simulink subsystem "Bat_lookup_2024a"  (R2024a)
settings: Solver=VariableStepAuto  StartTime=0.0  StopTime=10.0  RelTol=1e-3
settings Model: Creator=User  LastModifiedBy=User

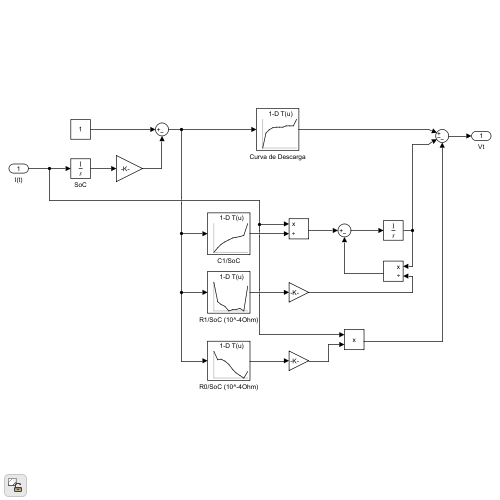
[thumbnail: Simulink's stored preview of the top-level diagram]
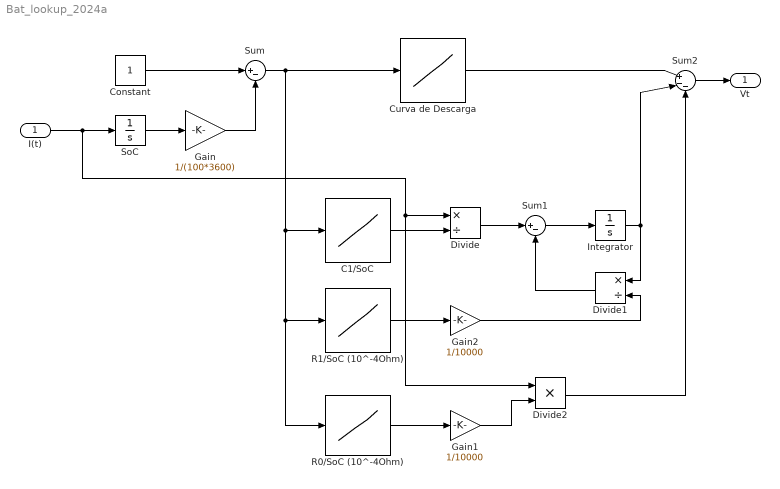
== system Bat_lookup_2024a ==
  I(t) : Inport
  C1/SoC : Lookup_n-D  NumberOfTableDimensions=1  BreakpointsForDimension1=[0.1;0.2;0.3;0.4;0.5;0.6;0.7;0.8;0.9;1]  Table=[14627;21365;25642;29230;32161;34533;36341;37291;38369;55644]  InternalRulePriority=Speed  RndMeth=Simplest
  Constant : Constant
  Curva de Descarga : Lookup_n-D  NumberOfTableDimensions=1  BreakpointsForDimension1=[0 0.10000000000000001 0.20000000000000001 0.29999999999999999 0.40000000000000002 0.5 0.59999999999999998 0.69999999999999996 0.80000000000000004 0.90000000000000002 1]  Table=[2.734 3.127 3.213 3.256 3.278 3.28 3.285 3.308 3.319 3.32 3.493]  InternalRulePriority=Speed  RndMeth=Simplest
  Divide : Product  Inputs=*/
  Divide1 : Product  Inputs=*/
  Divide2 : Product  Inputs=**
  Gain : Gain  Gain=1/(100*3600)
  Gain1 : Gain  Gain=1/10000
  Gain2 : Gain  Gain=1/10000
  Integrator : Integrator
  R0/SoC (10^-4Ohm) : Lookup_n-D  NumberOfTableDimensions=1  BreakpointsForDimension1=[0.1;0.2;0.3;0.4;0.5;0.6;0.7;0.8;0.9;1]  Table=[9.364100000000001;8.653499999999999;8.7011;8.558;8.243;7.82;7.545;7.324;7.073;7.6313]  InternalRulePriority=Speed  RndMeth=Simplest
  R1/SoC (10^-4Ohm) : Lookup_n-D  NumberOfTableDimensions=1  BreakpointsForDimension1=[0.1;0.2;0.3;0.4;0.5;0.6;0.7;0.8;0.9;1]  Table=[8.720000000000001;5.2166;4.764;4.438;3.66;3.8324;3.8639;4.0732;3.6497;7.949]  InternalRulePriority=Speed  RndMeth=Simplest
  SoC : Integrator
  Sum : Sum  Inputs=|+-
  Sum1 : Sum  Inputs=|+-
  Sum2 : Sum  Inputs=|+--
  Vt : Outport
  wires:
  I(t)/1 -> SoC/1, Divide/1, Divide2/1
  C1/SoC/1 -> Divide/2
  Divide/1 -> Sum1/1
  Sum1/1 -> Integrator/1
  Integrator/1 -> Sum2/2, Divide1/1
  R1/SoC (10^-4Ohm)/1 -> Gain2/1
  Divide1/1 -> Sum1/2
  Sum2/1 -> Vt/1
  Curva de Descarga/1 -> Sum2/1
  Divide2/1 -> Sum2/3
  R0/SoC (10^-4Ohm)/1 -> Gain1/1
  Gain2/1 -> Divide1/2
  Gain1/1 -> Divide2/2
  SoC/1 -> Gain/1
  Gain/1 -> Sum/2
  Constant/1 -> Sum/1
  Sum/1 -> R0/SoC (10^-4Ohm)/1, R1/SoC (10^-4Ohm)/1, C1/SoC/1, Curva de Descarga/1
